simulink model "task_1"  (R2024a)
settings: Solver=VariableStepAuto  StartTime=0.0  StopTime=30.0  RelTol=1e-3
settings Model: Creator=alexe  LastModifiedBy=alexe

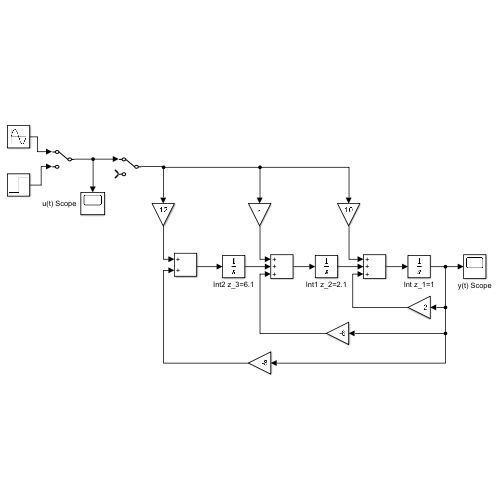
[thumbnail: Simulink's stored preview of the top-level diagram]
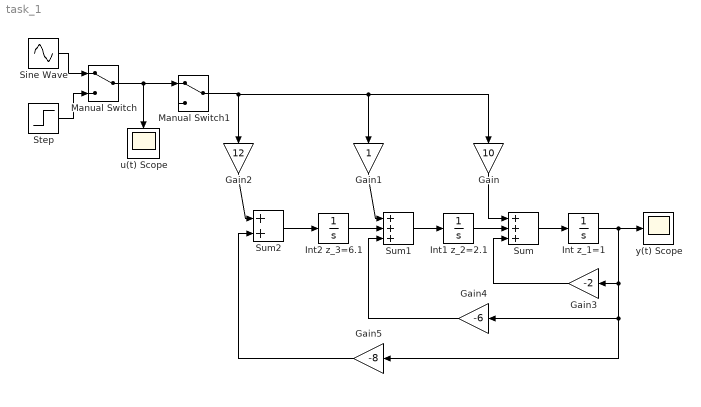
== system task_1 ==
  Gain : Gain  Gain=10
  Gain1 : Gain
  Gain2 : Gain  Gain=12
  Gain3 : Gain  Gain=-2
  Gain4 : Gain  Gain=-6
  Gain5 : Gain  Gain=-8
  Int z_1=1 : Integrator
  Int1 z_2=2.1 : Integrator
  Int2 z_3=6.1 : Integrator
  Manual Switch : ManualSwitch
  Manual Switch1 : ManualSwitch
  Sine Wave : Sin  Amplitude=2  SampleTime=0
  Step : Step  SampleTime=0
  Sum : Sum  Inputs=+++
  Sum1 : Sum  Inputs=+++
  Sum2 : Sum
  u(t) Scope : Scope
  y(t) Scope : Scope
  wires:
  Manual Switch1/1 -> Gain2/1, Gain/1, Gain1/1
  Gain2/1 -> Sum2/1
  Sum2/1 -> Int2 z_3=6.1/1
  Int2 z_3=6.1/1 -> Sum1/2
  Gain1/1 -> Sum1/1
  Sum1/1 -> Int1 z_2=2.1/1
  Gain/1 -> Sum/1
  Int1 z_2=2.1/1 -> Sum/2
  Sum/1 -> Int z_1=1/1
  Int z_1=1/1 -> Gain5/1, Gain4/1, Gain3/1, y(t) Scope/1
  Gain3/1 -> Sum/3
  Gain4/1 -> Sum1/3
  Gain5/1 -> Sum2/2
  Sine Wave/1 -> Manual Switch/1
  Step/1 -> Manual Switch/2
  Manual Switch/1 -> u(t) Scope/1, Manual Switch1/1
